simulink model "modello"  (R2025b)
settings: Solver=ode3  StartTime=0.0  StopTime=10.0  FixedStep=0.01  RelTol=1e-3
values from neighbouring files (symbols this model uses):
  MixerMatrix = [ 1/(4*Ct_eq), -1/(4*Ct_eq*Drone.L), -1/(4*Ct_eq*Drone.L),  1/(4*Cq_eq) ... (first row only)    [test_track.m]
  rho = 1.225    [test_track.m]
undefined symbols (not defined in the file or in its folder): bounds, Drone, dyn_obs, max_angular_vel, max_deviazione_pos, max_distanza_goal, max_vel, num_rays, PID, pos_goal, tolleranza_goal
libraries: slpidlib x6, matrix_library x2, rllib x1
settings Model: Creator=gabri  LastModifiedBy=gabri

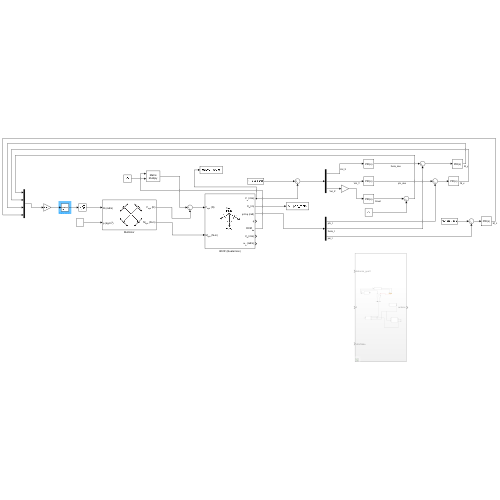
[thumbnail: Simulink's stored preview of the top-level diagram]
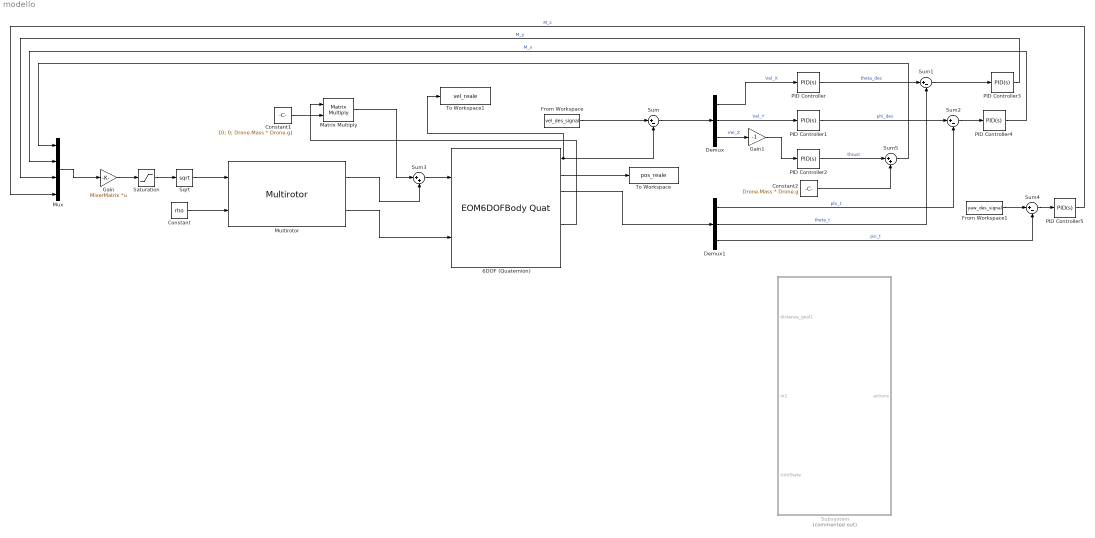
== system modello ==
  6DOF (Quaternion) : EOM6DOFBodyQuat  mass_0=Drone.Mass  inertia=Drone.Inertia
  Constant : Constant  Value=rho
  Constant1 : Constant  Value=[0; 0; Drone.Mass * Drone.g]
  Constant2 : Constant  Value=Drone.Mass * Drone.g
  Demux : Demux  Outputs=3
  Demux1 : Demux  Outputs=3
  From Workspace : FromWorkspace  VariableName=vel_des_signal
  From Workspace1 : FromWorkspace  VariableName=yaw_des_signal
  Gain : Gain  Gain=MixerMatrix  Multiplication=Matrix(K*u)
  Gain1 : Gain  Gain=-1
  Matrix Multiply : Product  Multiplication=Matrix(*)
  Multirotor : Multirotor  armLength=Drone.L  rotorHeight=0.01  CT=Drone.Ct  CQ=Drone.Cq  radius=Drone.Radius
  Mux : Mux
  PID Controller : slpidlib/PID Controller  Controller=PID  Form=Parallel  TimeDomain=Continuous-time  UseExternalTs=off  SampleTime=-1  IntegratorMethod=Forward Euler  FilterMethod=Forward Euler  ControllerParametersSource=internal  P=PID.XY_Kp  I=PID.XY_Ki  UseKiTs=off  D=PID.XY_Kd  UseExternalDerivativeSource=off  N=100  UseFilter=on  TunerSelectOption=Transfer Function Based (PID Tuner App)  InitialConditionSource=internal  InitialConditionForIntegrator=0  InitialConditionForFilter=0  DifferentiatorICPrevScaledInput=0  ExternalReset=none  TrackingMode=off  Kt=1  LimitOutput=off  SatLimitsSource=internal  UpperSaturationLimit=inf  LowerSaturationLimit=-inf  LinearizeAsGain=on  AntiWindupMode=none  Kb=1  LimitIntegrator=off  UpperIntegratorSaturationLimit=inf  LowerIntegratorSaturationLimit=-inf  POutMin=[]  POutMax=[]  IOutMin=[]  IOutMax=[]  DOutMin=[]  DOutMax=[]  NOutMin=[]  NOutMax=[]  SumOutMin=[]  SumOutMax=[]  SaturationOutMin=[]  SaturationOutMax=[]  PParamMin=[]  PParamMax=[]  IParamMin=[]  IParamMax=[]  DParamMin=[]  DParamMax=[]  NParamMin=[]  NParamMax=[]  KbParamMin=[]  KbParamMax=[]  KtParamMin=[]  KtParamMax=[]  KbOutMin=[]  KbOutMax=[]  KtOutMin=[]  KtOutMax=[]  IntegratorOutMin=[]  IntegratorOutMax=[]  FilterOutMin=[]  FilterOutMax=[]  SumI1OutMin=[]  SumI1OutMax=[]  SumI2OutMin=[]  SumI2OutMax=[]  SumI3OutMin=[]  SumI3OutMax=[]  SumI4OutMin=[]  SumI4OutMax=[]  SumDOutMin=[]  SumDOutMax=[]  DifferentiatorOutMin=[]  DifferentiatorOutMax=[]  FilterDiffOutCoefMin=[]  FilterDiffOutCoefMax=[]  ReciprocalOutMin=[]  ReciprocalOutMax=[]  SumDenOutMin=[]  SumDenOutMax=[]  SumNumOutMin=[]  SumNumOutMax=[]  DivideOutMin=[]  DivideOutMax=[]  UdiffTsProdOutMin=[]  UdiffTsProdOutMax=[]  NTsProdOutMin=[]  NTsProdOutMax=[]  UintegralTsProdOutMin=[]  UintegralTsProdOutMax=[]  UngainTsProdOutMin=[]  UngainTsProdOutMax=[]  ClampingZeroOutDataTypeStr=Inherit: Inherit via back propagation  ClampingZeroOutMin=[]  ClampingZeroOutMax=[]  FilterDenConstantOutDataTypeStr=Inherit: Inherit via back propagation  FilterDenConstantOutMin=[]  FilterDenConstantOutMax=[]  PCopyOutDataTypeStr=Inherit: Inherit via back propagation  PCopyOutMin=[]  PCopyOutMax=[]  NCopyOutDataTypeStr=Inherit: Inherit via back propagation  NCopyOutMin=[]  NCopyOutMax=[]  IntegratorContinuousStateAttributes=''  IntegratorStateMustResolveToSignalObject=off  IntegratorRTWStateStorageClass=Auto  FilterContinuousStateAttributes=''  FilterStateMustResolveToSignalObject=off  FilterRTWStateStorageClass=Auto  ParallelPVariant=InternalParameters  IdealPVariant=Disabled  IVariant=InternalParameters  DVariant=InternalParameters  IntegratorVariant=Continuous  SatVariant=Disabled  AWVariant=Passthrough  PCopyVariant=Disabled  TRVariant=Disabled  FdbkBlocksVariant=Forward  IdealPFdbkVariant=Disabled  SatFdbkVariant=Disabled  DerivativeFilterVariant=ContFilter  NVariant=InternalParameters  NCopyVariant=Disabled  FilterICVariant=InternalICsFilter  IntegratorICVariant=InternalICs  ExternalResetVariant=Disabled  TRSumVariant=Passthrough  SumFdbkVariant=Disabled  SumVariant=Sum_PID  TsampFilterVariant=InternalTs  TsampNgainVariant=Passthrough  TsampIntegralVariant=Disabled_SignalSpec  ExternalSaturationOutDataTypeStr=Inherit: Same as second input  DerivativeSourceVariant=ErrorSignal  PreIntVariant=InternalPreInt
  PID Controller1 : slpidlib/PID Controller  Controller=PID  Form=Parallel  TimeDomain=Continuous-time  UseExternalTs=off  SampleTime=-1  IntegratorMethod=Forward Euler  FilterMethod=Forward Euler  ControllerParametersSource=internal  P=PID.XY_Kp  I=PID.XY_Ki  UseKiTs=off  D=PID.XY_Kd  UseExternalDerivativeSource=off  N=100  UseFilter=on  TunerSelectOption=Transfer Function Based (PID Tuner App)  InitialConditionSource=internal  InitialConditionForIntegrator=0  InitialConditionForFilter=0  DifferentiatorICPrevScaledInput=0  ExternalReset=none  TrackingMode=off  Kt=1  LimitOutput=off  SatLimitsSource=internal  UpperSaturationLimit=inf  LowerSaturationLimit=-inf  LinearizeAsGain=on  AntiWindupMode=none  Kb=1  LimitIntegrator=off  UpperIntegratorSaturationLimit=inf  LowerIntegratorSaturationLimit=-inf  POutMin=[]  POutMax=[]  IOutMin=[]  IOutMax=[]  DOutMin=[]  DOutMax=[]  NOutMin=[]  NOutMax=[]  SumOutMin=[]  SumOutMax=[]  SaturationOutMin=[]  SaturationOutMax=[]  PParamMin=[]  PParamMax=[]  IParamMin=[]  IParamMax=[]  DParamMin=[]  DParamMax=[]  NParamMin=[]  NParamMax=[]  KbParamMin=[]  KbParamMax=[]  KtParamMin=[]  KtParamMax=[]  KbOutMin=[]  KbOutMax=[]  KtOutMin=[]  KtOutMax=[]  IntegratorOutMin=[]  IntegratorOutMax=[]  FilterOutMin=[]  FilterOutMax=[]  SumI1OutMin=[]  SumI1OutMax=[]  SumI2OutMin=[]  SumI2OutMax=[]  SumI3OutMin=[]  SumI3OutMax=[]  SumI4OutMin=[]  SumI4OutMax=[]  SumDOutMin=[]  SumDOutMax=[]  DifferentiatorOutMin=[]  DifferentiatorOutMax=[]  FilterDiffOutCoefMin=[]  FilterDiffOutCoefMax=[]  ReciprocalOutMin=[]  ReciprocalOutMax=[]  SumDenOutMin=[]  SumDenOutMax=[]  SumNumOutMin=[]  SumNumOutMax=[]  DivideOutMin=[]  DivideOutMax=[]  UdiffTsProdOutMin=[]  UdiffTsProdOutMax=[]  NTsProdOutMin=[]  NTsProdOutMax=[]  UintegralTsProdOutMin=[]  UintegralTsProdOutMax=[]  UngainTsProdOutMin=[]  UngainTsProdOutMax=[]  ClampingZeroOutDataTypeStr=Inherit: Inherit via back propagation  ClampingZeroOutMin=[]  ClampingZeroOutMax=[]  FilterDenConstantOutDataTypeStr=Inherit: Inherit via back propagation  FilterDenConstantOutMin=[]  FilterDenConstantOutMax=[]  PCopyOutDataTypeStr=Inherit: Inherit via back propagation  PCopyOutMin=[]  PCopyOutMax=[]  NCopyOutDataTypeStr=Inherit: Inherit via back propagation  NCopyOutMin=[]  NCopyOutMax=[]  IntegratorContinuousStateAttributes=''  IntegratorStateMustResolveToSignalObject=off  IntegratorRTWStateStorageClass=Auto  FilterContinuousStateAttributes=''  FilterStateMustResolveToSignalObject=off  FilterRTWStateStorageClass=Auto  ParallelPVariant=InternalParameters  IdealPVariant=Disabled  IVariant=InternalParameters  DVariant=InternalParameters  IntegratorVariant=Continuous  SatVariant=Disabled  AWVariant=Passthrough  PCopyVariant=Disabled  TRVariant=Disabled  FdbkBlocksVariant=Forward  IdealPFdbkVariant=Disabled  SatFdbkVariant=Disabled  DerivativeFilterVariant=ContFilter  NVariant=InternalParameters  NCopyVariant=Disabled  FilterICVariant=InternalICsFilter  IntegratorICVariant=InternalICs  ExternalResetVariant=Disabled  TRSumVariant=Passthrough  SumFdbkVariant=Disabled  SumVariant=Sum_PID  TsampFilterVariant=InternalTs  TsampNgainVariant=Passthrough  TsampIntegralVariant=Disabled_SignalSpec  ExternalSaturationOutDataTypeStr=Inherit: Same as second input  DerivativeSourceVariant=ErrorSignal  PreIntVariant=InternalPreInt
  PID Controller2 : slpidlib/PID Controller  Controller=PID  Form=Parallel  TimeDomain=Continuous-time  UseExternalTs=off  SampleTime=-1  IntegratorMethod=Forward Euler  FilterMethod=Forward Euler  ControllerParametersSource=internal  P=PID.Z_Kp  I=PID.Z_Ki  UseKiTs=off  D=PID.Z_Kd  UseExternalDerivativeSource=off  N=100  UseFilter=on  TunerSelectOption=Transfer Function Based (PID Tuner App)  InitialConditionSource=internal  InitialConditionForIntegrator=0  InitialConditionForFilter=0  DifferentiatorICPrevScaledInput=0  ExternalReset=none  TrackingMode=off  Kt=1  LimitOutput=off  SatLimitsSource=internal  UpperSaturationLimit=inf  LowerSaturationLimit=-inf  LinearizeAsGain=on  AntiWindupMode=none  Kb=1  LimitIntegrator=off  UpperIntegratorSaturationLimit=inf  LowerIntegratorSaturationLimit=-inf  POutMin=[]  POutMax=[]  IOutMin=[]  IOutMax=[]  DOutMin=[]  DOutMax=[]  NOutMin=[]  NOutMax=[]  SumOutMin=[]  SumOutMax=[]  SaturationOutMin=[]  SaturationOutMax=[]  PParamMin=[]  PParamMax=[]  IParamMin=[]  IParamMax=[]  DParamMin=[]  DParamMax=[]  NParamMin=[]  NParamMax=[]  KbParamMin=[]  KbParamMax=[]  KtParamMin=[]  KtParamMax=[]  KbOutMin=[]  KbOutMax=[]  KtOutMin=[]  KtOutMax=[]  IntegratorOutMin=[]  IntegratorOutMax=[]  FilterOutMin=[]  FilterOutMax=[]  SumI1OutMin=[]  SumI1OutMax=[]  SumI2OutMin=[]  SumI2OutMax=[]  SumI3OutMin=[]  SumI3OutMax=[]  SumI4OutMin=[]  SumI4OutMax=[]  SumDOutMin=[]  SumDOutMax=[]  DifferentiatorOutMin=[]  DifferentiatorOutMax=[]  FilterDiffOutCoefMin=[]  FilterDiffOutCoefMax=[]  ReciprocalOutMin=[]  ReciprocalOutMax=[]  SumDenOutMin=[]  SumDenOutMax=[]  SumNumOutMin=[]  SumNumOutMax=[]  DivideOutMin=[]  DivideOutMax=[]  UdiffTsProdOutMin=[]  UdiffTsProdOutMax=[]  NTsProdOutMin=[]  NTsProdOutMax=[]  UintegralTsProdOutMin=[]  UintegralTsProdOutMax=[]  UngainTsProdOutMin=[]  UngainTsProdOutMax=[]  ClampingZeroOutDataTypeStr=Inherit: Inherit via back propagation  ClampingZeroOutMin=[]  ClampingZeroOutMax=[]  FilterDenConstantOutDataTypeStr=Inherit: Inherit via back propagation  FilterDenConstantOutMin=[]  FilterDenConstantOutMax=[]  PCopyOutDataTypeStr=Inherit: Inherit via back propagation  PCopyOutMin=[]  PCopyOutMax=[]  NCopyOutDataTypeStr=Inherit: Inherit via back propagation  NCopyOutMin=[]  NCopyOutMax=[]  IntegratorContinuousStateAttributes=''  IntegratorStateMustResolveToSignalObject=off  IntegratorRTWStateStorageClass=Auto  FilterContinuousStateAttributes=''  FilterStateMustResolveToSignalObject=off  FilterRTWStateStorageClass=Auto  ParallelPVariant=InternalParameters  IdealPVariant=Disabled  IVariant=InternalParameters  DVariant=InternalParameters  IntegratorVariant=Continuous  SatVariant=Disabled  AWVariant=Passthrough  PCopyVariant=Disabled  TRVariant=Disabled  FdbkBlocksVariant=Forward  IdealPFdbkVariant=Disabled  SatFdbkVariant=Disabled  DerivativeFilterVariant=ContFilter  NVariant=InternalParameters  NCopyVariant=Disabled  FilterICVariant=InternalICsFilter  IntegratorICVariant=InternalICs  ExternalResetVariant=Disabled  TRSumVariant=Passthrough  SumFdbkVariant=Disabled  SumVariant=Sum_PID  TsampFilterVariant=InternalTs  TsampNgainVariant=Passthrough  TsampIntegralVariant=Disabled_SignalSpec  ExternalSaturationOutDataTypeStr=Inherit: Same as second input  DerivativeSourceVariant=ErrorSignal  PreIntVariant=InternalPreInt
  PID Controller3 : slpidlib/PID Controller  Controller=PID  Form=Parallel  TimeDomain=Continuous-time  UseExternalTs=off  SampleTime=-1  IntegratorMethod=Forward Euler  FilterMethod=Forward Euler  ControllerParametersSource=internal  P=PID.Att_Kp  I=PID.Att_Ki  UseKiTs=off  D=PID.Att_Kd  UseExternalDerivativeSource=off  N=100  UseFilter=on  TunerSelectOption=Transfer Function Based (PID Tuner App)  InitialConditionSource=internal  InitialConditionForIntegrator=0  InitialConditionForFilter=0  DifferentiatorICPrevScaledInput=0  ExternalReset=none  TrackingMode=off  Kt=1  LimitOutput=off  SatLimitsSource=internal  UpperSaturationLimit=inf  LowerSaturationLimit=-inf  LinearizeAsGain=on  AntiWindupMode=none  Kb=1  LimitIntegrator=off  UpperIntegratorSaturationLimit=inf  LowerIntegratorSaturationLimit=-inf  POutMin=[]  POutMax=[]  IOutMin=[]  IOutMax=[]  DOutMin=[]  DOutMax=[]  NOutMin=[]  NOutMax=[]  SumOutMin=[]  SumOutMax=[]  SaturationOutMin=[]  SaturationOutMax=[]  PParamMin=[]  PParamMax=[]  IParamMin=[]  IParamMax=[]  DParamMin=[]  DParamMax=[]  NParamMin=[]  NParamMax=[]  KbParamMin=[]  KbParamMax=[]  KtParamMin=[]  KtParamMax=[]  KbOutMin=[]  KbOutMax=[]  KtOutMin=[]  KtOutMax=[]  IntegratorOutMin=[]  IntegratorOutMax=[]  FilterOutMin=[]  FilterOutMax=[]  SumI1OutMin=[]  SumI1OutMax=[]  SumI2OutMin=[]  SumI2OutMax=[]  SumI3OutMin=[]  SumI3OutMax=[]  SumI4OutMin=[]  SumI4OutMax=[]  SumDOutMin=[]  SumDOutMax=[]  DifferentiatorOutMin=[]  DifferentiatorOutMax=[]  FilterDiffOutCoefMin=[]  FilterDiffOutCoefMax=[]  ReciprocalOutMin=[]  ReciprocalOutMax=[]  SumDenOutMin=[]  SumDenOutMax=[]  SumNumOutMin=[]  SumNumOutMax=[]  DivideOutMin=[]  DivideOutMax=[]  UdiffTsProdOutMin=[]  UdiffTsProdOutMax=[]  NTsProdOutMin=[]  NTsProdOutMax=[]  UintegralTsProdOutMin=[]  UintegralTsProdOutMax=[]  UngainTsProdOutMin=[]  UngainTsProdOutMax=[]  ClampingZeroOutDataTypeStr=Inherit: Inherit via back propagation  ClampingZeroOutMin=[]  ClampingZeroOutMax=[]  FilterDenConstantOutDataTypeStr=Inherit: Inherit via back propagation  FilterDenConstantOutMin=[]  FilterDenConstantOutMax=[]  PCopyOutDataTypeStr=Inherit: Inherit via back propagation  PCopyOutMin=[]  PCopyOutMax=[]  NCopyOutDataTypeStr=Inherit: Inherit via back propagation  NCopyOutMin=[]  NCopyOutMax=[]  IntegratorContinuousStateAttributes=''  IntegratorStateMustResolveToSignalObject=off  IntegratorRTWStateStorageClass=Auto  FilterContinuousStateAttributes=''  FilterStateMustResolveToSignalObject=off  FilterRTWStateStorageClass=Auto  ParallelPVariant=InternalParameters  IdealPVariant=Disabled  IVariant=InternalParameters  DVariant=InternalParameters  IntegratorVariant=Continuous  SatVariant=Disabled  AWVariant=Passthrough  PCopyVariant=Disabled  TRVariant=Disabled  FdbkBlocksVariant=Forward  IdealPFdbkVariant=Disabled  SatFdbkVariant=Disabled  DerivativeFilterVariant=ContFilter  NVariant=InternalParameters  NCopyVariant=Disabled  FilterICVariant=InternalICsFilter  IntegratorICVariant=InternalICs  ExternalResetVariant=Disabled  TRSumVariant=Passthrough  SumFdbkVariant=Disabled  SumVariant=Sum_PID  TsampFilterVariant=InternalTs  TsampNgainVariant=Passthrough  TsampIntegralVariant=Disabled_SignalSpec  ExternalSaturationOutDataTypeStr=Inherit: Same as second input  DerivativeSourceVariant=ErrorSignal  PreIntVariant=InternalPreInt
  PID Controller4 : slpidlib/PID Controller  Controller=PID  Form=Parallel  TimeDomain=Continuous-time  UseExternalTs=off  SampleTime=-1  IntegratorMethod=Forward Euler  FilterMethod=Forward Euler  ControllerParametersSource=internal  P=PID.Att_Kp  I=PID.Att_Ki  UseKiTs=off  D=PID.Att_Kd  UseExternalDerivativeSource=off  N=100  UseFilter=on  TunerSelectOption=Transfer Function Based (PID Tuner App)  InitialConditionSource=internal  InitialConditionForIntegrator=0  InitialConditionForFilter=0  DifferentiatorICPrevScaledInput=0  ExternalReset=none  TrackingMode=off  Kt=1  LimitOutput=off  SatLimitsSource=internal  UpperSaturationLimit=inf  LowerSaturationLimit=-inf  LinearizeAsGain=on  AntiWindupMode=none  Kb=1  LimitIntegrator=off  UpperIntegratorSaturationLimit=inf  LowerIntegratorSaturationLimit=-inf  POutMin=[]  POutMax=[]  IOutMin=[]  IOutMax=[]  DOutMin=[]  DOutMax=[]  NOutMin=[]  NOutMax=[]  SumOutMin=[]  SumOutMax=[]  SaturationOutMin=[]  SaturationOutMax=[]  PParamMin=[]  PParamMax=[]  IParamMin=[]  IParamMax=[]  DParamMin=[]  DParamMax=[]  NParamMin=[]  NParamMax=[]  KbParamMin=[]  KbParamMax=[]  KtParamMin=[]  KtParamMax=[]  KbOutMin=[]  KbOutMax=[]  KtOutMin=[]  KtOutMax=[]  IntegratorOutMin=[]  IntegratorOutMax=[]  FilterOutMin=[]  FilterOutMax=[]  SumI1OutMin=[]  SumI1OutMax=[]  SumI2OutMin=[]  SumI2OutMax=[]  SumI3OutMin=[]  SumI3OutMax=[]  SumI4OutMin=[]  SumI4OutMax=[]  SumDOutMin=[]  SumDOutMax=[]  DifferentiatorOutMin=[]  DifferentiatorOutMax=[]  FilterDiffOutCoefMin=[]  FilterDiffOutCoefMax=[]  ReciprocalOutMin=[]  ReciprocalOutMax=[]  SumDenOutMin=[]  SumDenOutMax=[]  SumNumOutMin=[]  SumNumOutMax=[]  DivideOutMin=[]  DivideOutMax=[]  UdiffTsProdOutMin=[]  UdiffTsProdOutMax=[]  NTsProdOutMin=[]  NTsProdOutMax=[]  UintegralTsProdOutMin=[]  UintegralTsProdOutMax=[]  UngainTsProdOutMin=[]  UngainTsProdOutMax=[]  ClampingZeroOutDataTypeStr=Inherit: Inherit via back propagation  ClampingZeroOutMin=[]  ClampingZeroOutMax=[]  FilterDenConstantOutDataTypeStr=Inherit: Inherit via back propagation  FilterDenConstantOutMin=[]  FilterDenConstantOutMax=[]  PCopyOutDataTypeStr=Inherit: Inherit via back propagation  PCopyOutMin=[]  PCopyOutMax=[]  NCopyOutDataTypeStr=Inherit: Inherit via back propagation  NCopyOutMin=[]  NCopyOutMax=[]  IntegratorContinuousStateAttributes=''  IntegratorStateMustResolveToSignalObject=off  IntegratorRTWStateStorageClass=Auto  FilterContinuousStateAttributes=''  FilterStateMustResolveToSignalObject=off  FilterRTWStateStorageClass=Auto  ParallelPVariant=InternalParameters  IdealPVariant=Disabled  IVariant=InternalParameters  DVariant=InternalParameters  IntegratorVariant=Continuous  SatVariant=Disabled  AWVariant=Passthrough  PCopyVariant=Disabled  TRVariant=Disabled  FdbkBlocksVariant=Forward  IdealPFdbkVariant=Disabled  SatFdbkVariant=Disabled  DerivativeFilterVariant=ContFilter  NVariant=InternalParameters  NCopyVariant=Disabled  FilterICVariant=InternalICsFilter  IntegratorICVariant=InternalICs  ExternalResetVariant=Disabled  TRSumVariant=Passthrough  SumFdbkVariant=Disabled  SumVariant=Sum_PID  TsampFilterVariant=InternalTs  TsampNgainVariant=Passthrough  TsampIntegralVariant=Disabled_SignalSpec  ExternalSaturationOutDataTypeStr=Inherit: Same as second input  DerivativeSourceVariant=ErrorSignal  PreIntVariant=InternalPreInt
  PID Controller5 : slpidlib/PID Controller  Controller=PID  Form=Parallel  TimeDomain=Continuous-time  UseExternalTs=off  SampleTime=-1  IntegratorMethod=Forward Euler  FilterMethod=Forward Euler  ControllerParametersSource=internal  P=PID.Yaw_Kp  I=PID.Yaw_Ki  UseKiTs=off  D=PID.Yaw_Kd  UseExternalDerivativeSource=off  N=100  UseFilter=on  TunerSelectOption=Transfer Function Based (PID Tuner App)  InitialConditionSource=internal  InitialConditionForIntegrator=0  InitialConditionForFilter=0  DifferentiatorICPrevScaledInput=0  ExternalReset=none  TrackingMode=off  Kt=1  LimitOutput=off  SatLimitsSource=internal  UpperSaturationLimit=inf  LowerSaturationLimit=-inf  LinearizeAsGain=on  AntiWindupMode=none  Kb=1  LimitIntegrator=off  UpperIntegratorSaturationLimit=inf  LowerIntegratorSaturationLimit=-inf  POutMin=[]  POutMax=[]  IOutMin=[]  IOutMax=[]  DOutMin=[]  DOutMax=[]  NOutMin=[]  NOutMax=[]  SumOutMin=[]  SumOutMax=[]  SaturationOutMin=[]  SaturationOutMax=[]  PParamMin=[]  PParamMax=[]  IParamMin=[]  IParamMax=[]  DParamMin=[]  DParamMax=[]  NParamMin=[]  NParamMax=[]  KbParamMin=[]  KbParamMax=[]  KtParamMin=[]  KtParamMax=[]  KbOutMin=[]  KbOutMax=[]  KtOutMin=[]  KtOutMax=[]  IntegratorOutMin=[]  IntegratorOutMax=[]  FilterOutMin=[]  FilterOutMax=[]  SumI1OutMin=[]  SumI1OutMax=[]  SumI2OutMin=[]  SumI2OutMax=[]  SumI3OutMin=[]  SumI3OutMax=[]  SumI4OutMin=[]  SumI4OutMax=[]  SumDOutMin=[]  SumDOutMax=[]  DifferentiatorOutMin=[]  DifferentiatorOutMax=[]  FilterDiffOutCoefMin=[]  FilterDiffOutCoefMax=[]  ReciprocalOutMin=[]  ReciprocalOutMax=[]  SumDenOutMin=[]  SumDenOutMax=[]  SumNumOutMin=[]  SumNumOutMax=[]  DivideOutMin=[]  DivideOutMax=[]  UdiffTsProdOutMin=[]  UdiffTsProdOutMax=[]  NTsProdOutMin=[]  NTsProdOutMax=[]  UintegralTsProdOutMin=[]  UintegralTsProdOutMax=[]  UngainTsProdOutMin=[]  UngainTsProdOutMax=[]  ClampingZeroOutDataTypeStr=Inherit: Inherit via back propagation  ClampingZeroOutMin=[]  ClampingZeroOutMax=[]  FilterDenConstantOutDataTypeStr=Inherit: Inherit via back propagation  FilterDenConstantOutMin=[]  FilterDenConstantOutMax=[]  PCopyOutDataTypeStr=Inherit: Inherit via back propagation  PCopyOutMin=[]  PCopyOutMax=[]  NCopyOutDataTypeStr=Inherit: Inherit via back propagation  NCopyOutMin=[]  NCopyOutMax=[]  IntegratorContinuousStateAttributes=''  IntegratorStateMustResolveToSignalObject=off  IntegratorRTWStateStorageClass=Auto  FilterContinuousStateAttributes=''  FilterStateMustResolveToSignalObject=off  FilterRTWStateStorageClass=Auto  ParallelPVariant=InternalParameters  IdealPVariant=Disabled  IVariant=InternalParameters  DVariant=InternalParameters  IntegratorVariant=Continuous  SatVariant=Disabled  AWVariant=Passthrough  PCopyVariant=Disabled  TRVariant=Disabled  FdbkBlocksVariant=Forward  IdealPFdbkVariant=Disabled  SatFdbkVariant=Disabled  DerivativeFilterVariant=ContFilter  NVariant=InternalParameters  NCopyVariant=Disabled  FilterICVariant=InternalICsFilter  IntegratorICVariant=InternalICs  ExternalResetVariant=Disabled  TRSumVariant=Passthrough  SumFdbkVariant=Disabled  SumVariant=Sum_PID  TsampFilterVariant=InternalTs  TsampNgainVariant=Passthrough  TsampIntegralVariant=Disabled_SignalSpec  ExternalSaturationOutDataTypeStr=Inherit: Same as second input  DerivativeSourceVariant=ErrorSignal  PreIntVariant=InternalPreInt
  Saturation : Saturate  UpperLimit=inf  LowerLimit=1e-4
  Sqrt : Sqrt
  Subsystem : Subsystem  Commented=on
  Sum{,1..2,4} (4 alike) : Sum  Inputs=|+-
  Sum3 : Sum  Inputs=|++
  Sum5 : Sum  Inputs=|++
  To Workspace : ToWorkspace  VariableName=pos_reale  SampleTime=-1
  To Workspace1 : ToWorkspace  VariableName=vel_reale  SampleTime=-1
  wires:
  Multirotor/2 -> 6DOF (Quaternion)/2
  Constant/1 -> Multirotor/2
  From Workspace/1 -> Sum/1
  6DOF (Quaternion)/1 -> To Workspace1/1, Sum/2
  Sum/1 -> Demux/1
  Demux/1 -> PID Controller/1  "Vel_X"
  Demux/2 -> PID Controller1/1  "Vel_Y"
  Demux/3 -> Gain1/1  "Vel_Z"
  PID Controller/1 -> Sum1/1  "theta_des"
  6DOF (Quaternion)/3 -> Demux1/1
  Demux1/1 -> Sum2/2  "phi_t"
  PID Controller1/1 -> Sum2/1  "phi_des"
  PID Controller2/1 -> Sum5/1  "thrust"
  Demux1/3 -> Sum4/2  "psi_t"
  From Workspace1/1 -> Sum4/1
  Sqrt/1 -> Multirotor/1
  Gain/1 -> Saturation/1
  Mux/1 -> Gain/1
  Sum1/1 -> PID Controller3/1
  Sum2/1 -> PID Controller4/1
  Sum4/1 -> PID Controller5/1
  PID Controller4/1 -> Mux/2  "M_x"
  PID Controller5/1 -> Mux/4  "M_z"
  Demux1/2 -> Sum1/2  "theta_t"
  PID Controller3/1 -> Mux/3  "M_y"
  Saturation/1 -> Sqrt/1
  6DOF (Quaternion)/2 -> To Workspace/1
  6DOF (Quaternion)/5 -> Matrix Multiply/1
  Constant1/1 -> Matrix Multiply/2
  Multirotor/1 -> Sum3/2
  Matrix Multiply/1 -> Sum3/1
  Sum3/1 -> 6DOF (Quaternion)/1
  Constant2/1 -> Sum5/2
  Sum5/1 -> Mux/1
  Gain1/1 -> PID Controller2/1

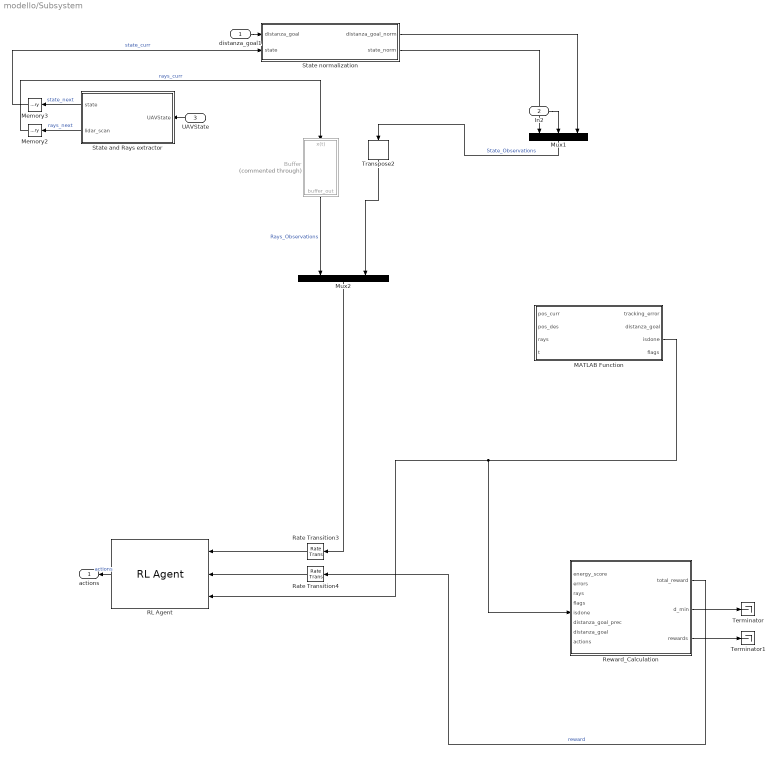
== system modello/Subsystem ==
  distanza_goal1 : Inport
  In2 : Inport  Port=2
  UAVState : Inport  Port=3
  Buffer : Subsystem  Commented=through
  MATLAB Function : MATLAB Function  TreatAsAtomicUnit=on
  Memory2 : Memory  InitialCondition=ones(1, num_rays)  InheritSampleTime=on  LinearizeMemory=on  LinearizeAsDelay=on
  Memory3 : Memory  InheritSampleTime=on  LinearizeMemory=on  LinearizeAsDelay=on
  Mux1 : Mux  Inputs=3
  Mux2 : Mux  Inputs=2
  RL Agent : rllib/RL Agent  Agent=agent  ExternalActionAsInput=off  ProvideLastAction=off  ProvideCumRwd=off  TreatAsDirectFeedthrough=on  UseStrictObservationDataTypes=off
  Rate Transition3 : RateTransition
  Rate Transition4 : RateTransition
  Reward_Calculation : MATLAB Function  TreatAsAtomicUnit=on
  State and Rays extractor : Subsystem
  State normalization : MATLAB Function  TreatAsAtomicUnit=on
  Terminator : Terminator
  Terminator1 : Terminator
  Transpose2 : matrix_library/Transpose
  actions : Outport
  wires:
  Memory3/1 -> State normalization/2(state)  "state_curr"
  State normalization/1(distanza_goal_norm) -> Mux1/3
  State and Rays extractor/1(state) -> Memory3/1  "state_next"
  State normalization/2(state_norm) -> Mux1/1
  Mux1/1 -> Transpose2/1  "State_Observations"
  Reward_Calculation/1(total_reward) -> Rate Transition4/1  "reward"
  Rate Transition4/1 -> RL Agent/2
  MATLAB Function/3(isdone) -> Reward_Calculation/5(isdone), RL Agent/3
  State and Rays extractor/2(lidar_scan) -> Memory2/1  "rays_next"
  Rate Transition3/1 -> RL Agent/1
  Mux2/1 -> Rate Transition3/1
  Buffer/1(buffer_out) -> Mux2/1  "Rays_Observations"
  Transpose2/1 -> Mux2/2
  Memory2/1 -> Buffer/1(x(t))  "rays_curr"
  UAVState/1 -> State and Rays extractor/1(UAVState)
  Reward_Calculation/3(rewards) -> Terminator1/1
  RL Agent/1 -> actions/1  "actions"
  distanza_goal1/1 -> State normalization/1(distanza_goal)
  In2/1 -> Mux1/2
  Reward_Calculation/2(d_min) -> Terminator/1

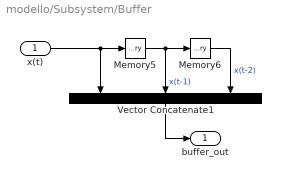
== system modello/Subsystem/Buffer ==
  x(t) : Inport
  Memory5 : Memory  InitialCondition=ones(1, num_rays)  InheritSampleTime=on  LinearizeMemory=on  LinearizeAsDelay=on
  Memory6 : Memory  InitialCondition=ones(1, num_rays)  InheritSampleTime=on  LinearizeMemory=on  LinearizeAsDelay=on
  Vector Concatenate1 : Concatenate  NumInputs=3
  buffer_out : Outport
  wires:
  Memory6/1 -> Vector Concatenate1/3  "x(t-2)"
  Memory5/1 -> Memory6/1, Vector Concatenate1/2  "x(t-1)"
  x(t)/1 -> Memory5/1, Vector Concatenate1/1
  Vector Concatenate1/1 -> buffer_out/1

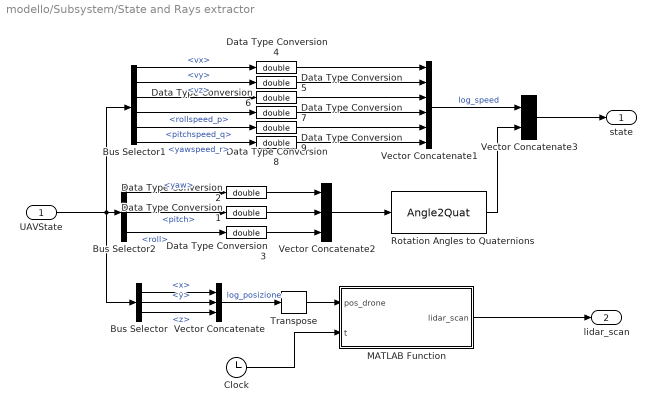
== system modello/Subsystem/State and Rays extractor ==
  UAVState : Inport
  Bus Selector : BusSelector  OutputSignals=pos_vel.x,pos_vel.y,pos_vel.z
  Bus Selector1 : BusSelector  OutputSignals=pos_vel.vx,pos_vel.vy,pos_vel.vz,attitude.rollspeed_p,attitude.pitchspeed_q,attitude.yawspeed_r
  Bus Selector2 : BusSelector  OutputSignals=attitude.yaw,attitude.pitch,attitude.roll
  Clock : Clock
  Data Type Conversion{1..9} (9 alike) : DataTypeConversion  OutDataTypeStr=double  SaturateOnIntegerOverflow=off  RndMeth=Floor
  MATLAB Function : MATLAB Function  TreatAsAtomicUnit=on
  Rotation Angles to Quaternions : Angle2Quat
      settings: AttributesFormatString=Rotation Order: %<rotationOrder>
  Transpose : matrix_library/Transpose
  Vector Concatenate : Concatenate  NumInputs=3
  Vector Concatenate1 : Concatenate  NumInputs=6
  Vector Concatenate2 : Concatenate  NumInputs=3
  Vector Concatenate3 : Concatenate
  state : Outport  OutDataTypeStr=double
  lidar_scan : Outport  Port=2  OutDataTypeStr=double
  wires:
  Vector Concatenate1/1 -> Vector Concatenate3/1  "log_speed"
  Bus Selector1/1 -> Data Type Conversion4/1  "<vx>"
  Rotation Angles to Quaternions/1 -> Vector Concatenate3/2
  Bus Selector1/4 -> Data Type Conversion7/1  "<rollspeed_p>"
  UAVState/1 -> Bus Selector2/1, Bus Selector/1, Bus Selector1/1
  Bus Selector1/2 -> Data Type Conversion5/1  "<vy>"
  Bus Selector1/5 -> Data Type Conversion8/1  "<pitchspeed_q>"
  Vector Concatenate/1 -> Transpose/1  "log_posizione"
  Bus Selector/1 -> Vector Concatenate/1  "<x>"
  Bus Selector1/3 -> Data Type Conversion6/1  "<vz>"
  Bus Selector1/6 -> Data Type Conversion9/1  "<yawspeed_r>"
  Vector Concatenate2/1 -> Rotation Angles to Quaternions/1
  Bus Selector/3 -> Vector Concatenate/3  "<z>"
  Bus Selector/2 -> Vector Concatenate/2  "<y>"
  Vector Concatenate3/1 -> state/1
  Bus Selector2/2 -> Data Type Conversion1/1  "<pitch>"
  Data Type Conversion1/1 -> Vector Concatenate2/2
  Bus Selector2/1 -> Data Type Conversion2/1  "<yaw>"
  Data Type Conversion2/1 -> Vector Concatenate2/1
  Data Type Conversion3/1 -> Vector Concatenate2/3
  Bus Selector2/3 -> Data Type Conversion3/1  "<roll>"
  Data Type Conversion4/1 -> Vector Concatenate1/1
  Data Type Conversion5/1 -> Vector Concatenate1/2
  Data Type Conversion6/1 -> Vector Concatenate1/3
  Data Type Conversion7/1 -> Vector Concatenate1/4
  Data Type Conversion8/1 -> Vector Concatenate1/5
  Data Type Conversion9/1 -> Vector Concatenate1/6
  Transpose/1 -> MATLAB Function/1(pos_drone)
  Clock/1 -> MATLAB Function/2(t)
  MATLAB Function/1(lidar_scan) -> lidar_scan/1

== matlab function modello/Subsystem/State and Rays extractor/MATLAB Function ==
  data: pos_drone input; lidar_scan output double; bounds parameter; dyn_obs parameter; t input; num_rays parameter
function lidar_scan = estrai_lidar_scan(pos_drone, bounds, dyn_obs, t, num_rays)
    % Parametri del sensore
    max_range = 20.0; % Raggio massimo in metri
    % Aumentiamo i raggi: 256 o 512 sono buoni compromessi per RL in 3D
    
    % === 1. GENERAZIONE DIREZIONI RAGGI (SFERA DI FIBONACCI) ===
    % Genera vettori direzione unitari uniformemente distribuiti in 3D.
    indices = 0:(num_rays - 1);
    phi = pi * (3 - sqrt(5)); % Angolo aureo in radianti
    
    % La Z varia uniformemente da 1 (Polo Nord) a -1 (Polo Sud)
    z = 1 - (indices ./ (num_rays - 1)) .* 2; 
    
    % Raggio sul piano XY per l'altezza Z corrente
    raggio_xy = sqrt(1 - z.^2); 
    
    % Angolo di rotazione attorno all'asse Z
    theta = phi .* indices;      
    
    % Calcolo componenti X e Y
    x = cos(theta) .* raggio_xy;
    y = sin(theta) .* raggio_xy;
    
    % Matrice 3 x num_rays di vettori direzione unitari
    dirs = double([x; y; z]); 
    
    % Inizializza l'array delle misurazioni alla distanza massima
    lidar_scan = max_range * ones(1, num_rays, 'double');

    pos_drone = double(pos_drone);

    % === 1.5 ADATTAMENTO FORMATO BOUNDS (STRUCT o MATRICE) ===
    % Questo blocco rende la funzione universale per qualsiasi tipo di mappa
    if isstruct(bounds)
        b_xmin = bounds.x_min; b_xmax = bounds.x_max;
        b_ymin = bounds.y_min; b_ymax = bounds.y_max;
        b_zmin = bounds.z_min; b_zmax = bounds.z_max;
    else
        % Se bounds è una matrice Nx6 (es. map.v)
        if size(bounds, 2) >= 6
            % Controlla se il formato è [xmin, xmax, ymin, ymax, ...] o [xmin, ymin, zmin, xmax, ...]
            if bounds(1,2) > bounds(1,1) && bounds(1,4) > bounds(1,3)
                b_xmin = bounds(:,1); b_xmax = bounds(:,2);
                b_ymin = bounds(:,3); b_ymax = bounds(:,4);
                b_zmin = bounds(:,5); b_zmax = bounds(:,6);
            else
                b_xmin = bounds(:,1); b_xmax = bounds(:,4);
                b_ymin = bounds(:,2); b_ymax = bounds(:,5);
                b_zmin = bounds(:,3); b_zmax = bounds(:,6);
            end
        else
            b_xmin = []; b_xmax = []; b_ymin = []; b_ymax = []; b_zmin = []; b_zmax = [];
        end
    end

    % === 2. INTERSEZIONE CON OSTACOLI STATICI (PALAZZI - SLAB METHOD) ===
    if ~isempty(b_xmin)
        % Uso i vettori estratti al passo 1.5
        vicini_idx = find(~(b_xmax < pos_drone(1)-max_range | b_xmin > pos_drone(1)+max_range | ...
                            b_ymax < pos_drone(2)-max_range | b_ymin > pos_drone(2)+max_range | ...
                            b_zmax < pos_drone(3)-max_range | b_zmin > pos_drone(3)+max_range));

    % === 2. INTERSEZIONE CON OSTACOLI STATICI (PALAZZI - SLAB METHOD) ===
    vicini_idx = find(~(bounds.x_max < pos_drone(1)-max_range | bounds.x_min > pos_drone(1)+max_range | ...
                        bounds.y_max < pos_drone(2)-max_range | bounds.y_min > pos_drone(2)+max_range | ...
                        bounds.z_max < pos_drone(3)-max_range | bounds.z_min > pos_drone(3)+max_range));
                        
    if ~isempty(vicini_idx)
        % Precalcola i reciproci delle direzioni per lo Slab Method.
        % L'aggiunta di 1e-8 previene divisioni per zero quando un raggio 
        % è perfettamente parallelo a un asse.
        inv_dirs = 1 ./ (dirs + 1e-8); 
        
        for i = 1:length(vicini_idx)
            idx = vicini_idx(i);
            
            % Limiti del bounding box corrente
            b_min = [bounds.x_min(idx); bounds.y_min(idx); bounds.z_min(idx)];
            b_max = [bounds.x_max(idx); bounds.y_max(idx); bounds.z_max(idx)];
            
            % Calcola i tempi di intersezione con i piani min e max per gli assi XYZ
            % (Operazione matriciale 3 x num_rays)
            t0 = (b_min - pos_drone(:)) .* inv_dirs; 
            t1 = (b_max - pos_drone(:)) .* inv_dirs; 
            
            % tmin è il tempo di ingresso nel piano, tmax l'uscita per ogni asse
            tmin = min(t0, t1); 
            tmax = max(t0, t1); 
            
            % Il raggio entra nel box quando ha superato TUTTI E TRE i piani min
            t_enter = max(tmin, [], 1); % Estrae il max lungo le colonne (1 x num_rays)
            
            % Il raggio esce dal box appena supera UNO DEI TRE piani max
            t_exit = min(tmax, [], 1);  % Estrae il min lungo le colonne (1 x num_rays)
            
            % Condizione di intersezione Ray-AABB:
            % 1. Entra prima di uscire (t_enter <= t_exit)
            % 2. L'uscita è davanti al drone (t_exit > 0)
            hit_mask = (t_enter <= t_exit) & (t_exit > 0);
            
            if any(hit_mask)
                hitting_rays = find(hit_mask);
                for j = 1:length(hitting_rays)
                    r_idx = hitting_rays(j);
                    
                    % Se il drone è all'interno del palazzo, t_enter è negativo.
                    % In tal caso, la distanza di impatto è 0 (schianto istantaneo).
                    if t_enter(r_idx) > 0
                        d_imp = t_enter(r_idx);
                    else
                        d_imp = 0; 
                    end
                    
                    % Sovrascrivi se questo palazzo è più vicino di altri ostacoli già visti
                    if d_imp < lidar_scan(r_idx)
                        lidar_scan(r_idx) = d_imp;
                    end
                end
            end
        end
    end

    % === 3. INTERSEZIONE CON OSTACOLI DINAMICI (SFERE) ===
    if ~isempty(dyn_obs)
        for k = 1:length(dyn_obs)

            %Calcola la posizione attuale dell'ostacolo: P(t) = P0 + V*t
            centro_sfera = dyn_obs(k).p0 + dyn_obs(k).v * t;
            raggio_sfera = dyn_obs(k).radius;
            
            % Vettore dal drone al centro della sfera (3x1)
            v = centro_sfera(:) - pos_drone(:);
            
            % Proiezione vettorializzata: dot product tra 'v' e tutti i raggi 'dirs'
            proj = v' * dirs; 
            
            % Consideriamo solo i raggi per cui la sfera è "in avanti"
            valid_idx = proj > 0;
            
            if any(valid_idx)
                % Calcolo distanza ortogonale per i raggi validi
                distanza_ortogonale_sq = dot(v, v) - proj(valid_idx).^2;
                
                % Trova quali raggi hanno colpito la sfera
                hit_idx = distanza_ortogonale_sq <= raggio_sfera^2;
                
                if any(hit_idx)
                    actual_rays = find(valid_idx);
                    hitting_rays = actual_rays(hit_idx);
                    
                    proj_hits = proj(hitting_rays);
                    dist_ort_sq_hits = distanza_ortogonale_sq(hit_idx);
                    distanza_impatto = proj_hits - sqrt(raggio_sfera^2 - dist_ort_sq_hits);
                    
                    for i = 1:length(hitting_rays)
                        r_idx = hitting_rays(i);
                        d_imp = distanza_impatto(i);
                        if d_imp > 0 && d_imp < lidar_scan(r_idx)
                            lidar_scan(r_idx) = d_imp;
                        end
                    end
                end
            end
        end
    end

    % === 4. INTERSEZIONE CON IL TERRENO (PIANO Z = -1) ===
    % Consideriamo solo i raggi che puntano verso il basso (z < 0)
    downward_rays = dirs(3,:) < 0;

    if any(downward_rays)
        % Calcoliamo l'intersezione con il piano z=-0.5
        % L'equazione del piano è z = -0.5
        % Per un raggio con direzione (dx, dy, dz) e origine (x0, y0, z0):
        % z0 + t*dz = -0.5 => t = (-0.5 - z0)/dz
        t_ground = (-0.5 - pos_drone(3)) ./ dirs(3, downward_rays);

        % Filtriamo solo le intersezioni valide (t > 0)
        valid_ground = t_ground > 0;

        if any(valid_ground)
            ground_rays = find(downward_rays);
            valid_ground_rays = ground_rays(valid_ground);

            % Calcoliamo le distanze di impatto
            d_imp = t_ground(valid_ground);

            % Aggiorniamo le misurazioni lidar
            for i = 1:length(valid_ground_rays)
                r_idx = valid_ground_rays(i);
                if d_imp(i) < lidar_scan(r_idx)
                    lidar_scan(r_idx) = d_imp(i);
                end
            end
        end
    end
    
    % Normalizzazione
    % L'output è un array flat [1 x num_rays] con valori nel range [0, 1]
    lidar_scan = double(lidar_scan) / max_range;
end

== matlab function modello/Subsystem/MATLAB Function ==
  data: tracking_error output; distanza_goal output; pos_curr input; isdone output; pos_des input; rays input; pos_goal parameter size=[1 3]; flags output; t input; max_deviazione_pos parameter; tolleranza_goal parameter
function [tracking_error, distanza_goal, isdone, flags] = check_terminal_state(pos_curr, pos_des, rays, pos_goal, t, max_deviazione_pos, tolleranza_goal)

    persistent raggio_drone
    persistent soglia_impatto
    persistent max_range_raggi

    if isempty(raggio_drone)
   
        raggio_drone = 0.5; % Ingombro fisico del drone in metri (30 cm)
        max_range_raggi = 20; % Lo stesso usato nel raycasting
        soglia_impatto = raggio_drone / max_range_raggi;
    end

    pos_goal = pos_goal';


    % Ignora forzatamente il primo loop (t = 0)
    if t == 0
        isdone = false;
        flags = [false, false, false, false];
        distanza_goal = double(norm(pos_curr - pos_goal));
        tracking_error = 0;
        return; % Esce immediatamente dalla funzione
    end
    
    % 1. Controllo Divergenza (Tracking Error)
    % Calcola la distanza euclidea tra la posizione attuale e quella desiderata
    tracking_error = double(norm(pos_curr - pos_des));
    fuori_traiettoria =  tracking_error > max_deviazione_pos;
    
    % 2. Controllo Altitudine (Schianto a terra)
    % Presumendo che pos_curr(3) sia l'altitudine (asse Z positivo verso l'alto)
    quota_minima = 0;
    schianto_terra = pos_curr(3) < quota_minima;
    
    % 3. Controllo Collisione tramite raggi LiDAR
    % Si valuta se l'ostacolo più vicino penetra il raggio fisico del drone
    collisione = false;
    if min(rays) <= soglia_impatto
        collisione = true;
    end

    % Controllo Traguardo Raggiunto
    distanza_goal = double(norm(pos_curr - pos_goal));
    traguardo_raggiunto = distanza_goal < tolleranza_goal;

    flags = [fuori_traiettoria, schianto_terra, collisione, traguardo_raggiunto];
    
    % L'episodio termina se si verifica ALMENO UNA di queste condizioni
    isdone = fuori_traiettoria | schianto_terra | collisione | traguardo_raggiunto;
    
end

== matlab function modello/Subsystem/Reward_Calculation ==
  data: energy_score input; errors input; rays input; total_reward output; flags input; isdone input; distanza_goal_prec input; distanza_goal input; actions input; max_delta parameter; d_min output; rewards output
function [total_reward, d_min, rewards] = Reward_Calculation(energy_score, errors, rays, ...
    flags, isdone, distanza_goal_prec, distanza_goal, actions, max_delta)
    
    % persistent min_reward_deviazione max_reward_deviazione 
    % ... max_deviazione min_deviazione

    persistent soglia_energia usaDeen

    persistent peso_ostacoli peso_azioni peso_errore_deviazione_base ...
        peso_progresso peso_deen
    
    persistent penalty_crash reward_goal 

    persistent margine_ostacoli raggio_atterraggio max_moltiplicatore_deviazione

    d_min = -1;

    rewards = [0 0 0 0 0];
    
    % Inizializzazione costanti
    if isempty(peso_azioni)
        
        % imposta se usare il DEEN al posto della penalità per ostacoli
        usaDeen = false; 

        soglia_energia = -1200;

        margine_ostacoli = 1; % 100% del range lidar
        
        % -- Pesi reward --
        % peso_deen = 2.0;
        % peso_azioni = 4.0;
        % peso_ostacoli = 4;
        % peso_errore_deviazione_base = 1;
        % peso_progresso = 50;
        peso_deen = 1;
        peso_azioni = 5; %orig 1
        peso_ostacoli = 1;
        peso_progresso = 1; %orig 1
        peso_errore_deviazione_base = 1;
        
        % -- Parametri gain sheduling per atterraggio --
        raggio_atterraggio = 10.0; % Inizio frenata a 10 metri dal goal
        max_moltiplicatore_deviazione = 0; % orig 10.0 % Al goal, l'errore di deviazione è 10 volte più grave

        % -- Penalità terminali --
        % penalty_crash = -500;
        % reward_goal = 500;
        penalty_crash = -300;
        reward_goal = 300;
    end
    
    if isdone
        % ------------------------------------------------
        % REWARD TERMINALI
        % ------------------------------------------------
    
        % Inizializza il reward terminale a zero
        total_reward = 0;
        
        % Penalità se collisione, schianto o deviazione
        deviazione_eccessiva = flags(1);
        schianto_terra    = flags(2);
        collisione        = flags(3);
        
        if schianto_terra || collisione || deviazione_eccessiva
            total_reward = penalty_crash;
            return;
        end
        
        % Reward se raggiunge il goal
        traguardo_raggiunto = flags(4);
        
        if traguardo_raggiunto
            total_reward = reward_goal;
            return;
        end

        return;
    end

    % ------------------------------------------------
    % PENALITA' SU AZIONI
    % ------------------------------------------------
    % Norma L1. Forza l'agente verso l'output 0.
    azioni_pos = norm(actions(1:3));
    %azioni_vel = norm(actions(4:6));
    
    % La norma L2 massima per un vettore 3D è M * sqrt(3)
    max_norm_act_pos = max_delta(1) * sqrt(3);
    %max_norm_act_vel = max_delta(4) * sqrt(3);
    
    azione_pos_norm = norm(azioni_pos) / max_norm_act_pos;
    %azione_vel_norm = norm(azioni_vel) / max_norm_act_vel;
    
    % Media delle azioni, limitata a 1 (se l'agente viola i limiti per via del rumore)
    %azione_tot_norm = min((azione_pos_norm + azione_vel_norm) / 2, 1.0);

    %penalita_azioni = -peso_azioni * azione_tot_norm;

    penalita_azioni = -peso_azioni * azione_pos_norm;
    
    % ------------------------------------------------
    % PENALITA' PER OSTACOLI
    % ------------------------------------------------

    [penalita_ostacoli, d_min] = calc_obstacle_penalty(rays, peso_ostacoli, margine_ostacoli);

    % --------------------------------------------------------
    % PENALITA' DI TRACCIAMENTO
    % --------------------------------------------------------

    e_pos = norm(errors(1:3));
    e_vel = norm(errors(4:6));

    % Gain scheduling sugli errori

    peso_errore_deviazione = peso_errore_deviazione_base;

    %temporaneamente rimosso
    % if distanza_goal <= raggio_atterraggio
    %     peso_errore_deviazione = peso_errore_deviazione_base * ...
    %         (1 + (max_moltiplicatore_deviazione - 1) * ...
    %         ((raggio_atterraggio - distanza_goal) / raggio_atterraggio));
    % end
    
    penalita_errore_velocita = 0;
    % penalita_errore_velocita = -peso_errore_deviazione * e_vel;
    penalita_errore_posizione = -peso_errore_deviazione * e_pos;

    % ------------------------------------------------
    % CALCOLO PROGRESS REWARD
    % ------------------------------------------------
    
    avvicinamento = distanza_goal_prec - distanza_goal;

    if avvicinamento < 0
        avvicinamento = 0;
    end

    reward_progresso = peso_progresso * avvicinamento;
    
    % % Vettore spostamento reale del drone
    % v_reale = pos_corrente - pos_prec;
    % 
    % % Vettore spostamento desiderato (traiettoria nominale)
    % v_rif = pos_des - pos_des_prec;
    % 
    % % Normalizziamo il vettore di riferimento per ottenere solo la direzione
    % norma_v_rif = double(norm(v_rif));
    % 
    % if norma_v_rif > 1e-6
    %     dir_rif = v_rif / norma_v_rif;
    %     % Proiezione: quanti metri ha percorso il drone nella direzione GIUSTA?
    %     avanzamento = double(dot(v_reale, dir_rif));
    % 
    %     % Normalizziamo l'avanzamento rispetto a quello atteso per avere un valore ~[-1, 1]
    %     progresso_norm = avanzamento / norma_v_rif; 
    % else
    %     % Se la traiettoria di riferimento è ferma (es. hovering al goal)
    %     progresso_norm = 0.0; 
    % end
    % 
    % reward_progresso = peso_progresso * progresso_norm;
    
    % ------------------------------------------------
    % REWARD DEEN
    % ------------------------------------------------

    deen_output = energy_score;

    alpha = -0.1;
    reward_deen = alpha * (double(deen_output) - soglia_energia);
    reward_deen = min(reward_deen, 0);
    reward_deen = 1.0 - (1.0 / (1.0 + exp(reward_deen)));
    reward_deen = peso_deen * reward_deen;
    
    % total_reward = reward_deen * deen_scaling + terminal_reward ...
    %     + reward_deviazione * deviazione_scaling + survival_bonus;

    % ------------------------------------------------
    % REWARD TOTALE
    % ------------------------------------------------

    % rewards = [penalita_azioni penalita_ostacoli ...
    %     penalita_errore_posizione reward_deen reward_progresso];

    rewards = [penalita_azioni penalita_ostacoli ...
        penalita_errore_posizione penalita_errore_velocita reward_progresso];

    if usaDeen % si usa il DEEN al posto della penalità per ostacoli
        somma_pesi = peso_azioni +...
            peso_progresso + peso_deen + peso_errore_deviazione; %^2;
        somma_reward = penalita_azioni + ...
            penalita_errore_posizione + reward_deen + reward_progresso;
        total_reward = somma_reward / somma_pesi;

    else % si usa la penalità per ostacoli
        % somma_pesi = peso_azioni + peso_ostacoli + ...
        %     peso_progresso + peso_errore_deviazione; %^2;
        somma_reward = penalita_azioni + penalita_ostacoli + ...
            penalita_errore_posizione + reward_progresso + ...
            penalita_errore_velocita;
        total_reward = somma_reward;% / somma_pesi;
    end

    %total_reward = total_reward * 100;
    
end

function [r_obs, d_min] = calc_obstacle_penalty(lidar_scan_norm, w_o, d_safe, p)
    % calc_obstacle_penalty: Calcola la penalità in base alla distanza degli ostacoli
    %
    % INPUT:
    % lidar_scan_norm - Vettore lineare di distanze normalizzate (double)
    % w_o             - Peso massimo della penalità (scalare positivo)
    % d_safe          - Soglia di sicurezza (es. 0.25 = 25% del max_range)
    % p               - Grado del polinomio (di default 2 = repulsione quadratica)
    %
    % OUTPUT:
    % r_obs           - Penalità scalare negativa (o 0)

    if nargin < 4, p = 2; end

    % Trova l'ostacolo più vicino tra tutti i 256 raggi
    d_min = min(lidar_scan_norm);
    
    % Calcola la penalità solo se l'ostacolo ha superato la soglia di sicurezza
    if d_min < d_safe
        % Il termine (d_safe - d_min) / d_safe va da 0 (al limite di d_safe) a 1 (impatto)
        intensita = (d_safe - d_min) / d_safe;
        
        % Applica l'esponente e il peso (segno negativo perché è una penalità)
        r_obs = -w_o * (intensita ^ p);
    else
        r_obs = 0.0;
    end
end

== matlab function modello/Subsystem/State normalization ==
  data: distanza_goal_norm output; distanza_goal input; state input; state_norm output; max_angular_vel parameter; max_vel parameter; max_distanza_goal parameter
function [distanza_goal_norm, state_norm] = state_normalization(distanza_goal, state, max_angular_vel, max_vel, max_distanza_goal)
    vel = state(1:3);
    angular_vel = state(4:6);

    state_norm = state;

    vel_norm = vel / max_vel;
    angular_vel = angular_vel / max_angular_vel;

    vel_norm = max(min(vel_norm, 1.0), -1.0);
    angular_vel = max(min(angular_vel, 1.0), -1.0);

    state_norm(1:3) = vel_norm;
    state_norm(4:6) = angular_vel;

    distanza_goal_norm = distanza_goal / max_distanza_goal;
end
